simulink model "day3"  (R2017b)
settings: Solver=FixedStepAuto  StartTime=0.0  StopTime=1  FixedStep=0.002  RelTol=1e-3
libraries: simulink x4
settings Model: Creator=Admin  LastModifiedBy=Admin

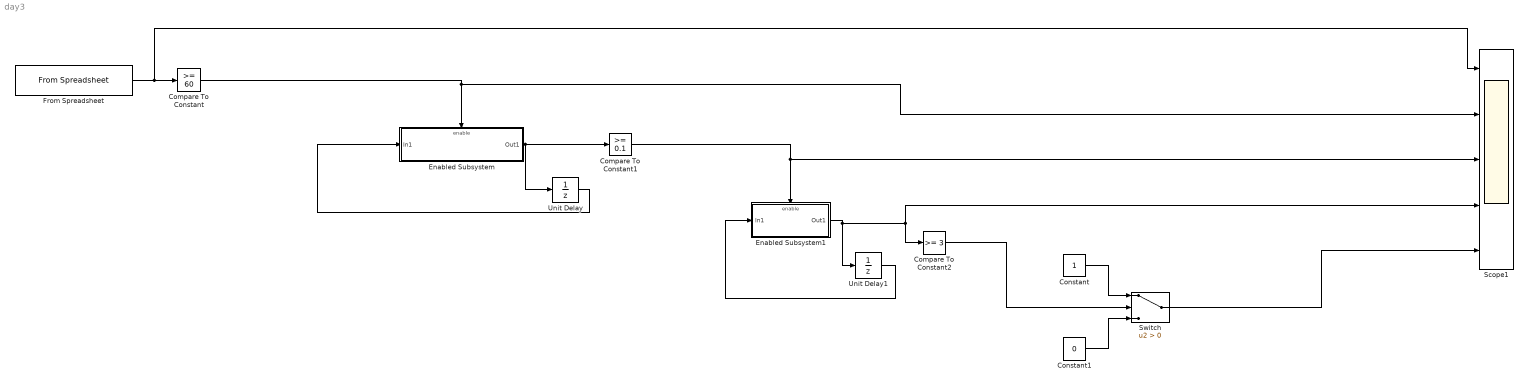
== system day3 ==
  Compare To Constant : simulink/Logic and Bit Operations/Compare To Constant  relop=>=  const=60  OutDataTypeStr=boolean
  Compare To Constant1 : simulink/Logic and Bit Operations/Compare To Constant  relop=>=  const=0.1  OutDataTypeStr=boolean
  Compare To Constant2 : simulink/Logic and Bit Operations/Compare To Constant  relop=>=  const=3  OutDataTypeStr=boolean
  Constant : Constant
  Constant1 : Constant  Value=0
  Enabled Subsystem : Subsystem  TreatAsAtomicUnit=on
  Enabled Subsystem1 : Subsystem  TreatAsAtomicUnit=on
  From Spreadsheet : FromSpreadsheet  FileName=dulieu.xlsx  SheetName=Sheet2
  Scope1 : Scope  NumInputPorts=5
  Switch : Switch  Criteria=u2 > Threshold
  Unit Delay : UnitDelay  SampleTime=-1
  Unit Delay1 : UnitDelay  SampleTime=-1
  wires:
  Compare To Constant/1 -> Scope1/2, Enabled Subsystem/Enable
  Enabled Subsystem/1(Out1) -> Unit Delay/1, Compare To Constant1/1
  Unit Delay/1 -> Enabled Subsystem/1(In1)
  Constant/1 -> Switch/1
  Constant1/1 -> Switch/3
  Switch/1 -> Scope1/5
  From Spreadsheet/1 -> Scope1/1, Compare To Constant/1
  Compare To Constant1/1 -> Enabled Subsystem1/Enable, Scope1/3
  Enabled Subsystem1/1(Out1) -> Compare To Constant2/1, Scope1/4, Unit Delay1/1
  Unit Delay1/1 -> Enabled Subsystem1/1(In1)
  Compare To Constant2/1 -> Switch/2

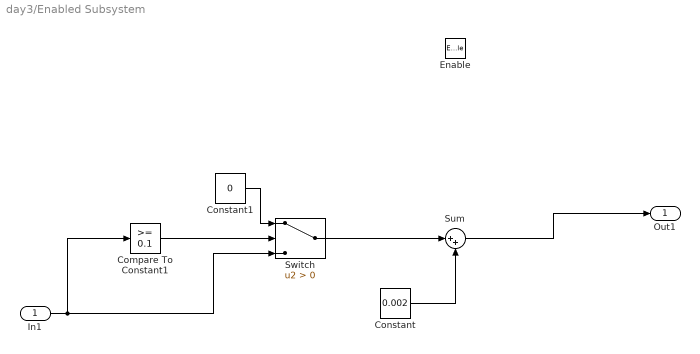
== system day3/Enabled Subsystem ==
  In1 : Inport
  Enable : EnablePort  StatesWhenEnabling=reset
  Compare To Constant1 : simulink/Logic and Bit Operations/Compare To Constant  relop=>=  const=0.1  OutDataTypeStr=boolean
  Constant : Constant  Value=0.002
  Constant1 : Constant  Value=0
  Sum : Sum  Inputs=|++
  Switch : Switch  Criteria=u2 > Threshold
  Out1 : Outport  OutputWhenDisabled=reset  InitialOutput=0
  wires:
  Constant/1 -> Sum/2
  Sum/1 -> Out1/1
  In1/1 -> Compare To Constant1/1, Switch/3
  Constant1/1 -> Switch/1
  Switch/1 -> Sum/1
  Compare To Constant1/1 -> Switch/2

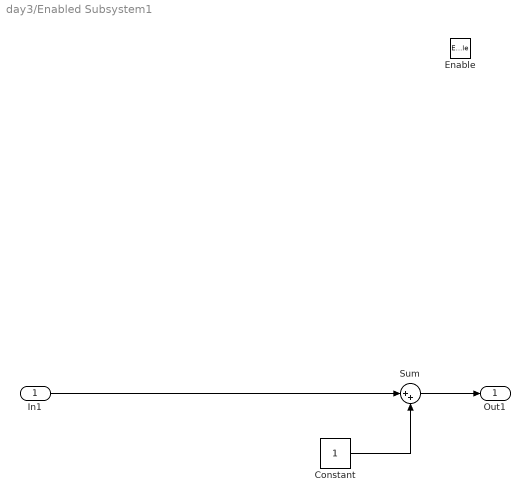
== system day3/Enabled Subsystem1 ==
  In1 : Inport
  Enable : EnablePort
  Constant : Constant
  Sum : Sum  Inputs=|++
  Out1 : Outport  InitialOutput=0
  wires:
  In1/1 -> Sum/1
  Constant/1 -> Sum/2
  Sum/1 -> Out1/1
